simulink model "drawingboard"  (R2019a)
settings: Solver=VariableStepAuto  StartTime=0.0  StopTime=2  RelTol=1e-3
settings Model: Creator=JanAriel  LastModifiedBy=JanAriel

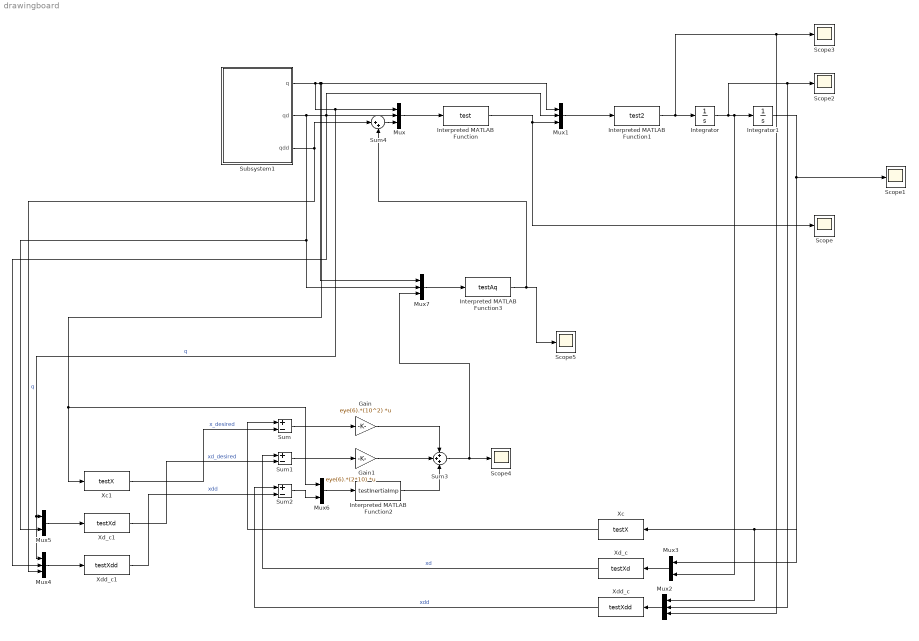
== system drawingboard ==
  Gain : Gain  Gain=eye(6).*(10^2)  Multiplication=Matrix(K*u) (u vector)
  Gain1 : Gain  Gain=eye(6).*(2*10)  Multiplication=Matrix(K*u) (u vector)
  Integrator : Integrator
  Integrator1 : Integrator
  Interpreted MATLAB Function : MATLABFcn  MATLABFcn=test
  Interpreted MATLAB Function1 : MATLABFcn  MATLABFcn=test2  Output1D=off
  Interpreted MATLAB Function2 : MATLABFcn  MATLABFcn=testInertiaImp  Output1D=off
  Interpreted MATLAB Function3 : MATLABFcn  MATLABFcn=testAq
  Mux{,1..2,4,7} (5 alike) : Mux  Inputs=3
  Mux3 : Mux  Inputs=2
  Mux5 : Mux  Inputs=2
  Mux6 : Mux  Inputs=2
  Scope{,1..5} (6 alike) : Scope
  Subsystem1 : Subsystem
  Sum : Sum  Inputs=+-
  Sum1 : Sum  Inputs=+-
  Sum2 : Sum  Inputs=+-
  Sum3 : Sum  Inputs=+++
  Sum4 : Sum  Inputs=|++
  Xc : MATLABFcn  MATLABFcn=testX
  Xc1 : MATLABFcn  MATLABFcn=testX
  Xd_c : MATLABFcn  MATLABFcn=testXd
  Xd_c1 : MATLABFcn  MATLABFcn=testXd
  Xdd_c : MATLABFcn  MATLABFcn=testXdd  Output1D=off
  Xdd_c1 : MATLABFcn  MATLABFcn=testXdd  Output1D=off
  wires:
  Subsystem1/1(q) -> Mux1/1, Mux6/1, Xc1/1, Mux7/1, Mux5/1, Mux4/1, Mux/1  "q"
  Subsystem1/3(qdd) -> Sum4/1, Mux4/3  "q"
  Mux/1 -> Interpreted MATLAB Function/1
  Interpreted MATLAB Function/1 -> Mux1/3, Scope/1
  Interpreted MATLAB Function1/1 -> Mux2/3, Scope3/1, Integrator/1
  Mux1/1 -> Interpreted MATLAB Function1/1
  Integrator/1 -> Mux3/2, Integrator1/1, Mux2/2, Scope2/1
  Integrator1/1 -> Mux3/1, Xc/1, Mux2/1, Scope1/1
  Mux2/1 -> Xdd_c/1
  Mux3/1 -> Xd_c/1
  Subsystem1/2(qd) -> Mux5/2, Mux7/2, Mux4/2, Mux1/2, Mux/2
  Mux4/1 -> Xdd_c1/1
  Mux5/1 -> Xd_c1/1
  Xc1/1 -> Sum/2  "x_desired"
  Xd_c1/1 -> Sum1/2  "xd_desired"
  Xd_c/1 -> Sum1/1  "xd"
  Xc/1 -> Sum/1
  Sum/1 -> Gain/1
  Sum1/1 -> Gain1/1
  Xdd_c/1 -> Sum2/1  "xdd"
  Xdd_c1/1 -> Sum2/2  "xdd"
  Gain1/1 -> Sum3/2
  Gain/1 -> Sum3/1
  Interpreted MATLAB Function2/1 -> Sum3/3
  Sum3/1 -> Mux7/3, Scope4/1
  Sum2/1 -> Mux6/2
  Mux6/1 -> Interpreted MATLAB Function2/1
  Interpreted MATLAB Function3/1 -> Scope5/1, Sum4/2
  Mux7/1 -> Interpreted MATLAB Function3/1
  Sum4/1 -> Mux/3

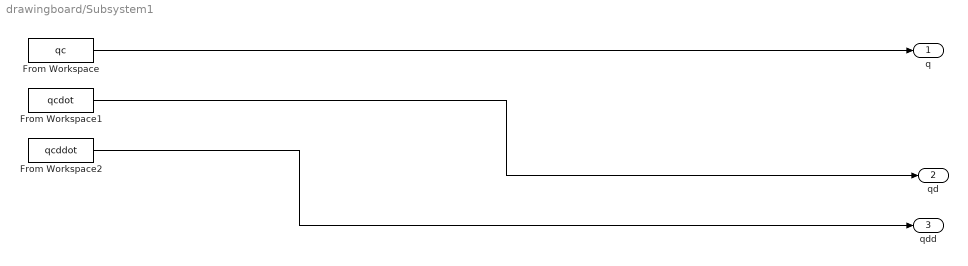
== system drawingboard/Subsystem1 ==
  From Workspace : FromWorkspace  VariableName=qc  SampleTime=0
  From Workspace1 : FromWorkspace  VariableName=qcdot  SampleTime=0
  From Workspace2 : FromWorkspace  VariableName=qcddot  SampleTime=0
  q : Outport
  qd : Outport  Port=2
  qdd : Outport  Port=3
  wires:
  From Workspace/1 -> q/1
  From Workspace1/1 -> qd/1
  From Workspace2/1 -> qdd/1
